simulink model "quad_control_elev8"  (Simulink 8.7)
settings: Solver=FixedStepAuto  StartTime=0.0  StopTime=20  FixedStep=0.01  RelTol=1e-3
InitFcn:
  | % --- Inner loop gains --------
  | Kp_pitch = 2.5;Ki_pitch = 0.005;Kd_pitch = 0.5;
  | 
  | Kp_roll = 2.5;Ki_roll = 0.005;Kd_roll = 0.5;
  | 
  | Kp_yaw = 10;Ki_yaw = 0.003;Kd_yaw = 2;
  | % --------------------------
  | 
  | % --- Outer loop gains --------
  | %P_X = 3.25; I_X = 0.45; D_X = 2;
  | %P_Y = 2.75; I_Y = 0.35; D_Y = 4.75;
  | %P_Z = 6; I_Z = 0.1; D_Z = 2;
  | 
  | %versoes 2
  | %P_X = 5;I_X = 0.1;D_X = 2.4;
  | %P_Y = 5;I_Y = 0.1;D_Y = 2.8;;
  | %P_Z = 32I_Z = 0.5;D_Z = 5;
  | 
  | %versoes CARLA
  | P_X = 9.44;I_X = 0.23;D_X = 2.36;
  | P_Y = 9.33;I_Y = 0.18;D_Y = 1.54;
  | P_Z = 28.09;I_Z = 5.65;D_Z = 16.16;
  | 
  | % --------------------------
  | 
  | % --- Saturation limits --------
  | attit_upper_limit = 10;
  | attit_lower_limit = -10;
  | 
  | pos_upper_limit = 1;
  | pos_lower_limit = -1;
  | 
  | mvel_upper_limit = 30;
  | mvel_lower_limit = 5;
  | % --------------------------
  | 
  | %gera o valor do angulo
  | %aleatoreamente para o treinamendo
  | %de posicao
  | rand_ang = pi + (-pi-pi).*rand(1,1);
  | rand_altur = 1 + (3-1).*rand(1,1);
  | 
  | global clientID;
  | clientID=-1;
undefined symbols (not defined in the file or in its folder): Angular, Linear, sigbuilder_block
libraries: simulink_extras x4, dspsigops x4, robotlib x3, aerolibtransform2 x1
settings Model: Creator=kleber  LastModifiedBy=kleber
settings DataIOCC: LimitDataPoints=off
settings DebuggingCC: UnderspecifiedInitializationDetection=Simplified  MergeDetectMultiDrivingBlocksExec=error  SolverPrmCheckMsg=warning
settings ConfigComp: CovSFcnEnable=off

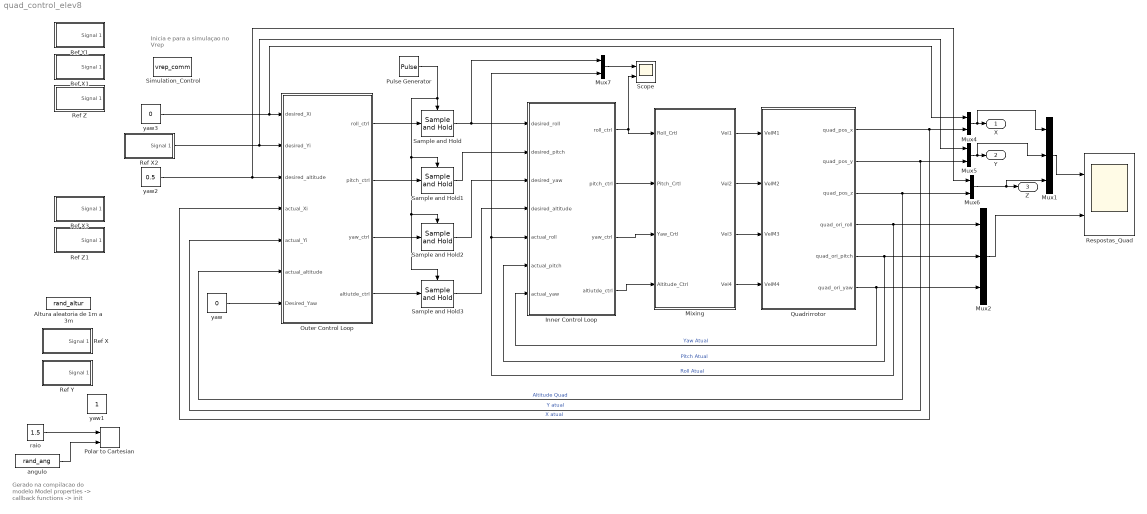
== system quad_control_elev8 ==
  note: Gerado na compilacao do modelo
      | Model properties -> callback functions
      | -> init
  note: Inicia e para a simulaçao no Vrep
  Altura aleatoria de 1m a 3m : Constant  Value=rand_altur
  Inner Control Loop : Subsystem
  Mixing : Subsystem
  Mux1 : Mux  Inputs=3
  Mux2 : Mux  Inputs=3
  Mux{4..7} (4 alike) : Mux  Inputs=2
  Outer Control Loop : Subsystem
  Polar to Cartesian : simulink_extras/Transformations/Polar to Cartesian
  Pulse Generator : DiscretePulseGenerator  PulseType=Time based  Period=0.1  PulseWidth=10
  Quadrirrotor : Subsystem
  Ref X : Subsystem  Tag=STV Subsys  LoadFcn=sigbuilder_block('load');  StartFcn=sigbuilder_block('start');  StopFcn=sigbuilder_block('stop');  ClipboardFcn=sigbuilder_block('clipboard');  mask(Sigbuilder block){}
      mask help: Sigbuilder GUI
      mask init:
      | if ~strcmp(get_param(bdroot(gcbh),'SimulationStatus'),'stopped') tuvar = sigbuilder_block('maskInit'); end
      settings: CopyFcn=sigbuilder_block('copy');  DeleteFcn=sigbuilder_block('delete');  ModelCloseFcn=sigbuilder_block('modelClose');  PreSaveFcn=sigbuilder_block('preSave');  PauseFcn=sigbuilder_block('pause')  ContinueFcn=sigbuilder_block('continue')  NameChangeFcn=sigbuilder_block('namechange');  OpenFcn=sigbuilder_block('open',[203.25 96 550.5 399.75 ]);  CloseFcn=sigbuilder_block('close');
      mask Display: plot(0,0,100,100,[10,10,40,40,10],[80,20,20,80,80],[40,10],[50,50], [40,27,10],[65,72,56],[40,25,25,10],[28,28,43,43]);
  Ref X1 : Subsystem  Tag=STV Subsys  LoadFcn=sigbuilder_block('load');  StartFcn=sigbuilder_block('start');  StopFcn=sigbuilder_block('stop');  ClipboardFcn=sigbuilder_block('clipboard');  mask(Sigbuilder block){}
      mask help: Sigbuilder GUI
      mask init:
      | if ~strcmp(get_param(bdroot(gcbh),'SimulationStatus'),'stopped') tuvar = sigbuilder_block('maskInit'); end
      settings: CopyFcn=sigbuilder_block('copy');  DeleteFcn=sigbuilder_block('delete');  ModelCloseFcn=sigbuilder_block('modelClose');  PreSaveFcn=sigbuilder_block('preSave');  PauseFcn=sigbuilder_block('pause')  ContinueFcn=sigbuilder_block('continue')  NameChangeFcn=sigbuilder_block('namechange');  OpenFcn=sigbuilder_block('open',[506.25 54.75 518.25 224.25 ]);  CloseFcn=sigbuilder_block('close');
      mask Display: plot(0,0,100,100,[10,10,40,40,10],[80,20,20,80,80],[40,10],[50,50], [40,27,10],[65,72,56],[40,25,25,10],[28,28,43,43]);
  Ref X2 : Subsystem  Tag=STV Subsys  LoadFcn=sigbuilder_block('load');  StartFcn=sigbuilder_block('start');  StopFcn=sigbuilder_block('stop');  ClipboardFcn=sigbuilder_block('clipboard');  mask(Sigbuilder block){}
      mask help: Sigbuilder GUI
      mask init:
      | if ~strcmp(get_param(bdroot(gcbh),'SimulationStatus'),'stopped') tuvar = sigbuilder_block('maskInit'); end
      settings: CopyFcn=sigbuilder_block('copy');  DeleteFcn=sigbuilder_block('delete');  ModelCloseFcn=sigbuilder_block('modelClose');  PreSaveFcn=sigbuilder_block('preSave');  PauseFcn=sigbuilder_block('pause')  ContinueFcn=sigbuilder_block('continue')  NameChangeFcn=sigbuilder_block('namechange');  OpenFcn=sigbuilder_block('open',[39.75 0 984.75 428.25 ]);  CloseFcn=sigbuilder_block('close');
      mask Display: plot(0,0,100,100,[10,10,40,40,10],[80,20,20,80,80],[40,10],[50,50], [40,27,10],[65,72,56],[40,25,25,10],[28,28,43,43]);
  Ref X3 : Subsystem  Tag=STV Subsys  LoadFcn=sigbuilder_block('load');  StartFcn=sigbuilder_block('start');  StopFcn=sigbuilder_block('stop');  ClipboardFcn=sigbuilder_block('clipboard');  mask(Sigbuilder block){}
      mask help: Sigbuilder GUI
      mask init:
      | if ~strcmp(get_param(bdroot(gcbh),'SimulationStatus'),'stopped') tuvar = sigbuilder_block('maskInit'); end
      settings: CopyFcn=sigbuilder_block('copy');  DeleteFcn=sigbuilder_block('delete');  ModelCloseFcn=sigbuilder_block('modelClose');  PreSaveFcn=sigbuilder_block('preSave');  PauseFcn=sigbuilder_block('pause')  ContinueFcn=sigbuilder_block('continue')  NameChangeFcn=sigbuilder_block('namechange');  OpenFcn=sigbuilder_block('open',[39.75 -17.25 984.75 495.75 ]);  CloseFcn=sigbuilder_block('close');
      mask Display: plot(0,0,100,100,[10,10,40,40,10],[80,20,20,80,80],[40,10],[50,50], [40,27,10],[65,72,56],[40,25,25,10],[28,28,43,43]);
  Ref Y : Subsystem  Tag=STV Subsys  LoadFcn=sigbuilder_block('load');  StartFcn=sigbuilder_block('start');  StopFcn=sigbuilder_block('stop');  ClipboardFcn=sigbuilder_block('clipboard');  mask(Sigbuilder block){}
      mask help: Sigbuilder GUI
      mask init:
      | if ~strcmp(get_param(bdroot(gcbh),'SimulationStatus'),'stopped') tuvar = sigbuilder_block('maskInit'); end
      settings: CopyFcn=sigbuilder_block('copy');  DeleteFcn=sigbuilder_block('delete');  ModelCloseFcn=sigbuilder_block('modelClose');  PreSaveFcn=sigbuilder_block('preSave');  PauseFcn=sigbuilder_block('pause')  ContinueFcn=sigbuilder_block('continue')  NameChangeFcn=sigbuilder_block('namechange');  OpenFcn=sigbuilder_block('open',[276 138 550.5 399.75 ]);  CloseFcn=sigbuilder_block('close');
      mask Display: plot(0,0,100,100,[10,10,40,40,10],[80,20,20,80,80],[40,10],[50,50], [40,27,10],[65,72,56],[40,25,25,10],[28,28,43,43]);
  Ref Y1 : Subsystem  Tag=STV Subsys  LoadFcn=sigbuilder_block('load');  StartFcn=sigbuilder_block('start');  StopFcn=sigbuilder_block('stop');  ClipboardFcn=sigbuilder_block('clipboard');  mask(Sigbuilder block){}
      mask help: Sigbuilder GUI
      mask init:
      | if ~strcmp(get_param(bdroot(gcbh),'SimulationStatus'),'stopped') tuvar = sigbuilder_block('maskInit'); end
      settings: CopyFcn=sigbuilder_block('copy');  DeleteFcn=sigbuilder_block('delete');  ModelCloseFcn=sigbuilder_block('modelClose');  PreSaveFcn=sigbuilder_block('preSave');  PauseFcn=sigbuilder_block('pause')  ContinueFcn=sigbuilder_block('continue')  NameChangeFcn=sigbuilder_block('namechange');  OpenFcn=sigbuilder_block('open',[270.75 145.5 510.75 222 ]);  CloseFcn=sigbuilder_block('close');
      mask Display: plot(0,0,100,100,[10,10,40,40,10],[80,20,20,80,80],[40,10],[50,50], [40,27,10],[65,72,56],[40,25,25,10],[28,28,43,43]);
  Ref Z : Subsystem  Tag=STV Subsys  LoadFcn=sigbuilder_block('load');  StartFcn=sigbuilder_block('start');  StopFcn=sigbuilder_block('stop');  ClipboardFcn=sigbuilder_block('clipboard');  mask(Sigbuilder block){}
      mask help: Sigbuilder GUI
      mask init:
      | if ~strcmp(get_param(bdroot(gcbh),'SimulationStatus'),'stopped') tuvar = sigbuilder_block('maskInit'); end
      settings: CopyFcn=sigbuilder_block('copy');  DeleteFcn=sigbuilder_block('delete');  ModelCloseFcn=sigbuilder_block('modelClose');  PreSaveFcn=sigbuilder_block('preSave');  PauseFcn=sigbuilder_block('pause')  ContinueFcn=sigbuilder_block('continue')  NameChangeFcn=sigbuilder_block('namechange');  OpenFcn=sigbuilder_block('open',[265.5 1.5 525.75 179.25 ]);  CloseFcn=sigbuilder_block('close');
      mask Display: plot(0,0,100,100,[10,10,40,40,10],[80,20,20,80,80],[40,10],[50,50], [40,27,10],[65,72,56],[40,25,25,10],[28,28,43,43]);
  Ref Z1 : Subsystem  Tag=STV Subsys  LoadFcn=sigbuilder_block('load');  StartFcn=sigbuilder_block('start');  StopFcn=sigbuilder_block('stop');  ClipboardFcn=sigbuilder_block('clipboard');  mask(Sigbuilder block){}
      mask help: Sigbuilder GUI
      mask init:
      | if ~strcmp(get_param(bdroot(gcbh),'SimulationStatus'),'stopped') tuvar = sigbuilder_block('maskInit'); end
      settings: CopyFcn=sigbuilder_block('copy');  DeleteFcn=sigbuilder_block('delete');  ModelCloseFcn=sigbuilder_block('modelClose');  PreSaveFcn=sigbuilder_block('preSave');  PauseFcn=sigbuilder_block('pause')  ContinueFcn=sigbuilder_block('continue')  NameChangeFcn=sigbuilder_block('namechange');  OpenFcn=sigbuilder_block('open',[58.5 0 966 213.75 ]);  CloseFcn=sigbuilder_block('close');
      mask Display: plot(0,0,100,100,[10,10,40,40,10],[80,20,20,80,80],[40,10],[50,50], [40,27,10],[65,72,56],[40,25,25,10],[28,28,43,43]);
  Respostas_Quad : Scope  NumInputPorts=2
  Sample and Hold{,1..3} (4 alike) : dspsigops/Sample and Hold  trig=Rising edge  initCond=0  latchinput=off
  Scope : Scope  NumInputPorts=2
  Simulation_Control : S-Function  FunctionName=vrep_comm  SFunctionDeploymentMode=off  EnableBusSupport=off
  angulo : Constant  Value=rand_ang
  raio : Constant  Value=1.5
  yaw : Constant  Value=0
  yaw1 : Constant
  yaw2 : Constant  Value=0.5
  yaw3 : Constant  Value=0
  X : Outport
  Y : Outport  Port=2
  Z : Outport  Port=3
  wires:
  Mux1/1 -> Respostas_Quad/1
  Mux2/1 -> Respostas_Quad/2
  Quadrirrotor/5(quad_ori_pitch) -> Inner Control Loop/6(actual_pitch), Mux2/2  "Pitch Atual"
  Quadrirrotor/4(quad_ori_roll) -> Mux7/2, Inner Control Loop/5(actual_roll), Mux2/1  "Roll Atual"
  Quadrirrotor/1(quad_pos_x) -> Outer Control Loop/4(actual_Xi), Mux4/2  "X atual"
  Quadrirrotor/3(quad_pos_z) -> Mux6/2, Outer Control Loop/6(actual_altitude)  "Altitude Quad"
  Quadrirrotor/6(quad_ori_yaw) -> Inner Control Loop/7(actual_yaw), Mux2/3  "Yaw Atual"
  Inner Control Loop/4(altiutde_ctrl) -> Mixing/4(Altitude_Ctrl)
  Sample and Hold3/1 -> Inner Control Loop/4(desired_altitude)
  Sample and Hold2/1 -> Inner Control Loop/3(desired_yaw)
  angulo/1 -> Polar to Cartesian/2
  raio/1 -> Polar to Cartesian/1
  yaw/1 -> Outer Control Loop/7(Desired_Yaw)
  Mux7/1 -> Scope/1
  Pulse Generator/1 -> Sample and Hold2/Trigger, Sample and Hold3/Trigger, Sample and Hold1/Trigger, Sample and Hold/Trigger
  Sample and Hold/1 -> Mux7/1, Inner Control Loop/1(desired_roll)
  Sample and Hold1/1 -> Inner Control Loop/2(desired_pitch)
  Outer Control Loop/4(altiutde_ctrl) -> Sample and Hold3/1
  Mux4/1 -> Mux1/1, X/1
  Mux5/1 -> Mux1/2, Y/1
  Mux6/1 -> Mux1/3, Z/1
  Ref X2/1(Signal 1) -> Mux5/1, Outer Control Loop/2(desired_Yi)
  yaw3/1 -> Mux4/1, Outer Control Loop/1(desired_Xi)
  yaw2/1 -> Mux6/1, Outer Control Loop/3(desired_altitude)
  Quadrirrotor/2(quad_pos_y) -> Outer Control Loop/5(actual_Yi), Mux5/2  "Y atual"
  Inner Control Loop/1(roll_ctrl) -> Mixing/1(Roll_Crtl), Scope/2
  Inner Control Loop/2(pitch_ctrl) -> Mixing/2(Pitch_Crtl)
  Inner Control Loop/3(yaw_ctrl) -> Mixing/3(Yaw_Crtl)
  Mixing/3(Vel3) -> Quadrirrotor/3(VelM3)
  Mixing/2(Vel2) -> Quadrirrotor/2(VelM2)
  Mixing/1(Vel1) -> Quadrirrotor/1(VelM1)
  Mixing/4(Vel4) -> Quadrirrotor/4(VelM4)
  Outer Control Loop/1(roll_ctrl) -> Sample and Hold/1
  Outer Control Loop/2(pitch_ctrl) -> Sample and Hold1/1
  Outer Control Loop/3(yaw_ctrl) -> Sample and Hold2/1

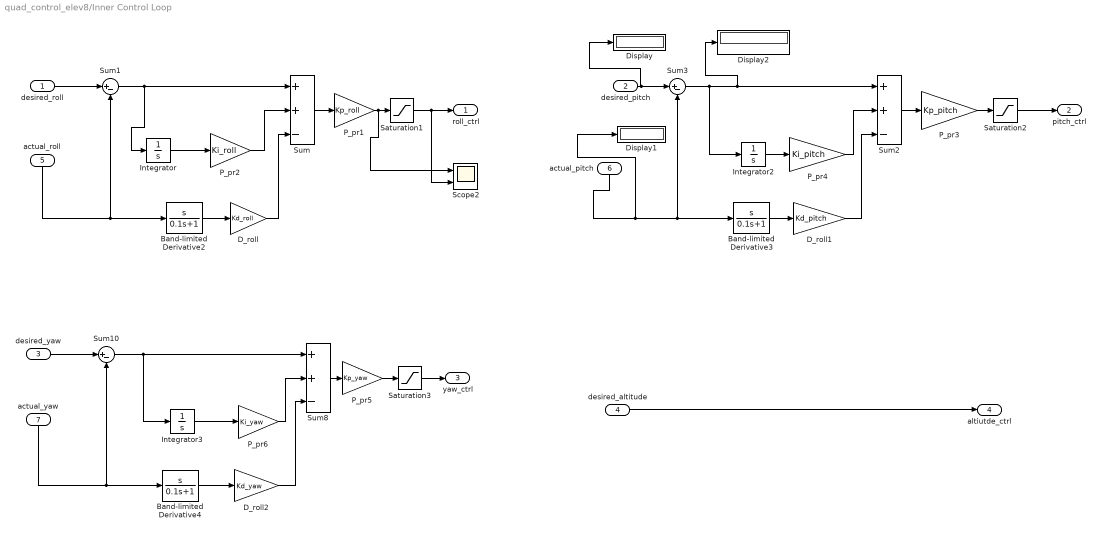
== system quad_control_elev8/Inner Control Loop ==
  desired_roll : Inport
  desired_pitch : Inport  Port=2
  desired_yaw : Inport  Port=3
  desired_altitude : Inport  Port=4
  actual_roll : Inport  Port=5
  actual_pitch : Inport  Port=6
  actual_yaw : Inport  Port=7
  Band-limited Derivative2 : TransferFcn  Numerator=[1 0]  Denominator=[0.1 1]
  Band-limited Derivative3 : TransferFcn  Numerator=[1 0]  Denominator=[0.1 1]
  Band-limited Derivative4 : TransferFcn  Numerator=[1 0]  Denominator=[0.1 1]
  D_roll : Gain  Gain=Kd_roll
  D_roll1 : Gain  Gain=Kd_pitch
  D_roll2 : Gain  Gain=Kd_yaw
  Display : Display
      settings: Decimation=3
  Display1 : Display
      settings: Decimation=3
  Display2 : Display
      settings: Decimation=3
  Integrator : Integrator
  Integrator2 : Integrator
  Integrator3 : Integrator
  P_pr1 : Gain  Gain=Kp_roll
  P_pr2 : Gain  Gain=Ki_roll
  P_pr3 : Gain  Gain=Kp_pitch
  P_pr4 : Gain  Gain=Ki_pitch
  P_pr5 : Gain  Gain=Kp_yaw
  P_pr6 : Gain  Gain=Ki_yaw
  Saturation1 : Saturate  UpperLimit=attit_upper_limit  LowerLimit=attit_lower_limit
  Saturation2 : Saturate  UpperLimit=attit_upper_limit  LowerLimit=attit_lower_limit
  Saturation3 : Saturate  UpperLimit=attit_upper_limit  LowerLimit=attit_lower_limit
  Scope2 : Scope  NumInputPorts=2
  Sum : Sum  Inputs=++-
  Sum1 : Sum  Inputs=|+-
  Sum10 : Sum  Inputs=|+-
  Sum2 : Sum  Inputs=++-
  Sum3 : Sum  Inputs=|+-
  Sum8 : Sum  Inputs=++-
  roll_ctrl : Outport
  pitch_ctrl : Outport  Port=2
  yaw_ctrl : Outport  Port=3
  altiutde_ctrl : Outport  Port=4
  wires:
  desired_altitude/1 -> altiutde_ctrl/1
  desired_roll/1 -> Sum1/1
  Sum1/1 -> Integrator/1, Sum/1
  Integrator/1 -> P_pr2/1
  actual_roll/1 -> Sum1/2, Band-limited Derivative2/1
  Band-limited Derivative2/1 -> D_roll/1
  desired_pitch/1 -> Display/1, Sum3/1
  Sum3/1 -> Sum2/1, Display2/1, Integrator2/1
  Integrator2/1 -> P_pr4/1
  actual_pitch/1 -> Sum3/2, Band-limited Derivative3/1, Display1/1
  Band-limited Derivative3/1 -> D_roll1/1
  desired_yaw/1 -> Sum10/1
  Sum10/1 -> Sum8/1, Integrator3/1
  Integrator3/1 -> P_pr6/1
  actual_yaw/1 -> Sum10/2, Band-limited Derivative4/1
  Band-limited Derivative4/1 -> D_roll2/1
  Saturation1/1 -> roll_ctrl/1, Scope2/2
  Saturation3/1 -> yaw_ctrl/1
  Saturation2/1 -> pitch_ctrl/1
  Sum/1 -> P_pr1/1
  P_pr1/1 -> Scope2/1, Saturation1/1
  D_roll/1 -> Sum/3
  D_roll1/1 -> Sum2/3
  Sum2/1 -> P_pr3/1
  P_pr3/1 -> Saturation2/1
  Sum8/1 -> P_pr5/1
  P_pr5/1 -> Saturation3/1
  D_roll2/1 -> Sum8/3
  P_pr2/1 -> Sum/2
  P_pr4/1 -> Sum2/2
  P_pr6/1 -> Sum8/2

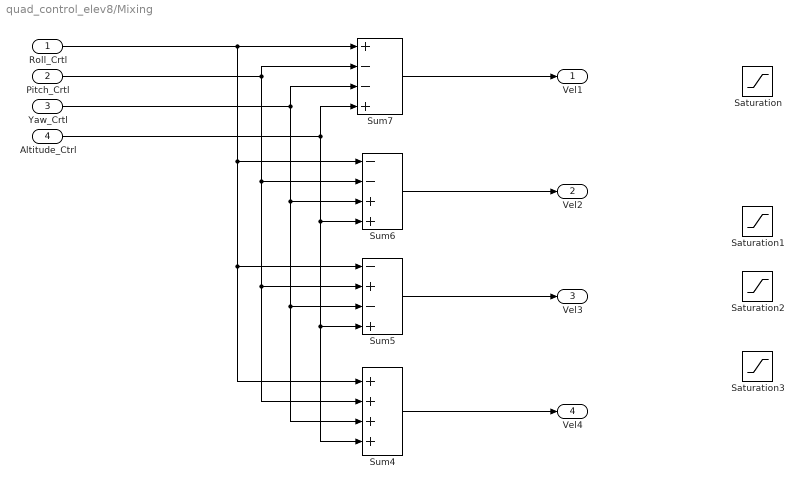
== system quad_control_elev8/Mixing ==
  Roll_Crtl : Inport
  Pitch_Crtl : Inport  Port=2
  Yaw_Crtl : Inport  Port=3
  Altitude_Ctrl : Inport  Port=4
  Saturation{,1..3} (4 alike) : Saturate  UpperLimit=mvel_upper_limit  LowerLimit=mvel_lower_limit
  Sum4 : Sum  Inputs=++++
  Sum5 : Sum  Inputs=-+-+
  Sum6 : Sum  Inputs=--++
  Sum7 : Sum  Inputs=+--+
  Vel1 : Outport
  Vel2 : Outport  Port=2
  Vel3 : Outport  Port=3
  Vel4 : Outport  Port=4
  wires:
  Yaw_Crtl/1 -> Sum4/3, Sum5/3, Sum6/3, Sum7/3
  Roll_Crtl/1 -> Sum4/1, Sum5/1, Sum6/1, Sum7/1
  Pitch_Crtl/1 -> Sum4/2, Sum5/2, Sum6/2, Sum7/2
  Altitude_Ctrl/1 -> Sum4/4, Sum5/4, Sum6/4, Sum7/4
  Sum7/1 -> Vel1/1
  Sum6/1 -> Vel2/1
  Sum5/1 -> Vel3/1
  Sum4/1 -> Vel4/1

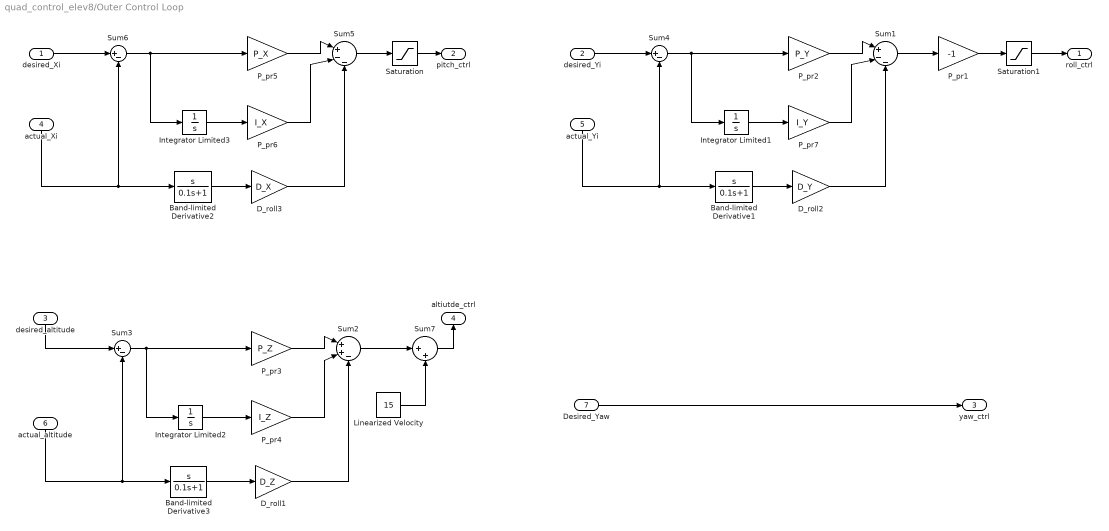
== system quad_control_elev8/Outer Control Loop ==
  desired_Xi : Inport
  desired_Yi : Inport  Port=2
  desired_altitude : Inport  Port=3
  actual_Xi : Inport  Port=4
  actual_Yi : Inport  Port=5
  actual_altitude : Inport  Port=6
  Desired_Yaw : Inport  Port=7
  Band-limited Derivative1 : TransferFcn  Numerator=[1 0]  Denominator=[0.1 1]
  Band-limited Derivative2 : TransferFcn  Numerator=[1 0]  Denominator=[0.1 1]
  Band-limited Derivative3 : TransferFcn  Numerator=[1 0]  Denominator=[0.1 1]
  D_roll1 : Gain  Gain=D_Z
  D_roll2 : Gain  Gain=D_Y
  D_roll3 : Gain  Gain=D_X
  Integrator Limited1 : Integrator  LimitOutput=on  UpperSaturationLimit=0.5  LowerSaturationLimit=-0.5
  Integrator Limited2 : Integrator  LimitOutput=on  UpperSaturationLimit=1  LowerSaturationLimit=0
  Integrator Limited3 : Integrator  LimitOutput=on  UpperSaturationLimit=0.5  LowerSaturationLimit=-0.5
  Linearized Velocity : Constant  Value=15
  P_pr1 : Gain  Gain=-1
  P_pr2 : Gain  Gain=P_Y
  P_pr3 : Gain  Gain=P_Z
  P_pr4 : Gain  Gain=I_Z
  P_pr5 : Gain  Gain=P_X
  P_pr6 : Gain  Gain=I_X
  P_pr7 : Gain  Gain=I_Y
  Saturation : Saturate  UpperLimit=2  LowerLimit=-2
  Saturation1 : Saturate  UpperLimit=2  LowerLimit=-2
  Sum1 : Sum  Inputs=|+--
  Sum2 : Sum  Inputs=|++-
  Sum3 : Sum  Inputs=|+-
  Sum4 : Sum  Inputs=|+-
  Sum5 : Sum  Inputs=|+--
  Sum6 : Sum  Inputs=|+-
  Sum7 : Sum  Inputs=|++
  roll_ctrl : Outport
  pitch_ctrl : Outport  Port=2
  yaw_ctrl : Outport  Port=3
  altiutde_ctrl : Outport  Port=4
  wires:
  Sum3/1 -> Integrator Limited2/1, P_pr3/1
  Integrator Limited2/1 -> P_pr4/1
  P_pr3/1 -> Sum2/1
  P_pr4/1 -> Sum2/2
  D_roll1/1 -> Sum2/3
  actual_altitude/1 -> Sum3/2, Band-limited Derivative3/1
  Band-limited Derivative3/1 -> D_roll1/1
  desired_altitude/1 -> Sum3/1
  Sum7/1 -> altiutde_ctrl/1
  Desired_Yaw/1 -> yaw_ctrl/1
  Sum6/1 -> Integrator Limited3/1, P_pr5/1
  Integrator Limited3/1 -> P_pr6/1
  P_pr5/1 -> Sum5/1
  D_roll3/1 -> Sum5/3
  actual_Xi/1 -> Band-limited Derivative2/1, Sum6/2
  Band-limited Derivative2/1 -> D_roll3/1
  desired_Xi/1 -> Sum6/1
  P_pr6/1 -> Sum5/2
  Sum4/1 -> Integrator Limited1/1, P_pr2/1
  Integrator Limited1/1 -> P_pr7/1
  P_pr2/1 -> Sum1/1
  D_roll2/1 -> Sum1/3
  actual_Yi/1 -> Band-limited Derivative1/1, Sum4/2
  Band-limited Derivative1/1 -> D_roll2/1
  desired_Yi/1 -> Sum4/1
  P_pr7/1 -> Sum1/2
  Sum1/1 -> P_pr1/1
  Sum2/1 -> Sum7/1
  Linearized Velocity/1 -> Sum7/2
  Sum5/1 -> Saturation/1
  Saturation/1 -> pitch_ctrl/1
  P_pr1/1 -> Saturation1/1
  Saturation1/1 -> roll_ctrl/1

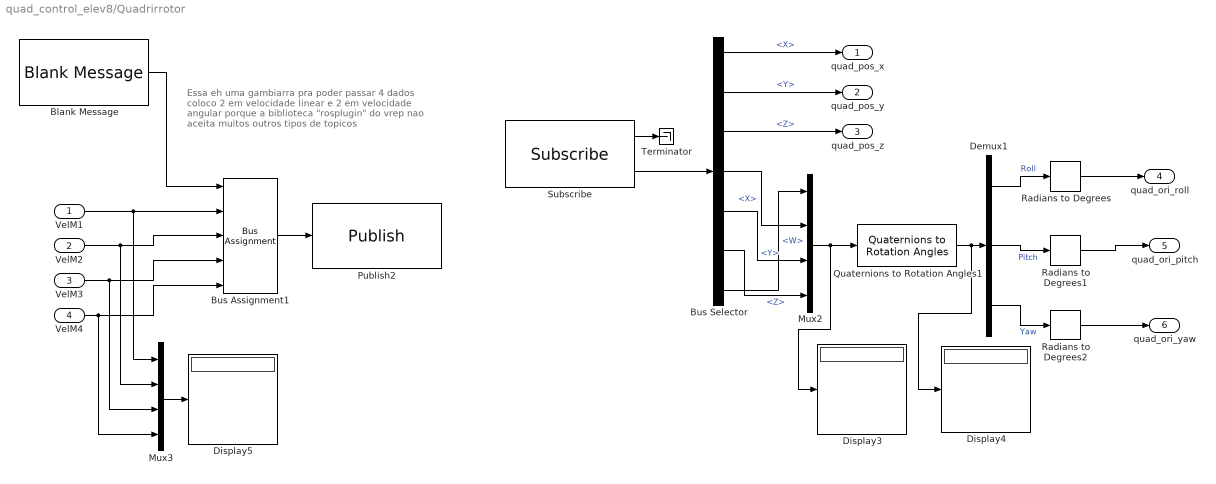
== system quad_control_elev8/Quadrirrotor ==
  note: Essa eh uma gambiarra pra poder passar 4 dados coloco 2 em velocidade linear e 2 em velocidade angular porque a biblioteca "rosplugin" do vrep nao aceita muitos outros tipos de topicos
  VelM1 : Inport
  VelM2 : Inport  Port=2
  VelM3 : Inport  Port=3
  VelM4 : Inport  Port=4
  Blank Message : robotlib/Blank Message  SourceLibraryInfo=This block requires Robotics System Toolbox  messageType=geometry_msgs/Twist  SampleTime=inf
  Bus Assignment1 : BusAssignment  DialogController=Simulink.DDGSource_BusAssignment  AssignedSignals=Linear.X,Linear.Y,Angular.X,Angular.Y
  Bus Selector : BusSelector  OutputSignals=Pose.Position.X,Pose.Position.Y,Pose.Position.Z,Pose.Orientation.X,Pose.Orientation.Y,Pose.Orientation.Z,Pose.Orientation.W
  Demux1 : Demux  Outputs=3
  Display3 : Display
  Display4 : Display
  Display5 : Display
  Mux2 : Mux
  Mux3 : Mux
  Publish2 : robotlib/Publish  SourceLibraryInfo=This block requires Robotics System Toolbox  topicSource=Select from ROS network  topic=/control_signals  messageType=geometry_msgs/Twist  messageQueueLength=105
  Quaternions to Rotation Angles1 : aerolibtransform2/Quaternions to Rotation Angles  rotationOrder=XYZ
  Radians to Degrees : simulink_extras/Transformations/Radians to Degrees
  Radians to Degrees1 : simulink_extras/Transformations/Radians to Degrees
  Radians to Degrees2 : simulink_extras/Transformations/Radians to Degrees
  Subscribe : robotlib/Subscribe  SourceLibraryInfo=This block requires Robotics System Toolbox  topicSource=Select from ROS network  topic=/quad_pos_ang  messageType=geometry_msgs/PoseStamped  sampleTime=-1  messageQueueLength=51
  Terminator : Terminator
  quad_pos_x : Outport
  quad_pos_y : Outport  Port=2
  quad_pos_z : Outport  Port=3
  quad_ori_roll : Outport  Port=4
  quad_ori_pitch : Outport  Port=5
  quad_ori_yaw : Outport  Port=6
  wires:
  VelM1/1 -> Mux3/1, Bus Assignment1/2
  Bus Selector/1 -> quad_pos_x/1  "<X>"
  Bus Selector/2 -> quad_pos_y/1  "<Y>"
  Bus Selector/3 -> quad_pos_z/1  "<Z>"
  Bus Assignment1/1 -> Publish2/1
  Blank Message/1 -> Bus Assignment1/1
  Subscribe/2 -> Bus Selector/1
  Subscribe/1 -> Terminator/1
  Bus Selector/5 -> Mux2/3  "<Y>"
  Bus Selector/6 -> Mux2/4  "<Z>"
  Bus Selector/7 -> Mux2/1  "<W>"
  Mux2/1 -> Quaternions to Rotation Angles1/1, Display3/1
  Bus Selector/4 -> Mux2/2  "<X>"
  VelM3/1 -> Mux3/3, Bus Assignment1/4
  VelM4/1 -> Mux3/4, Bus Assignment1/5
  Quaternions to Rotation Angles1/1 -> Display4/1, Demux1/1
  Mux3/1 -> Display5/1
  VelM2/1 -> Mux3/2, Bus Assignment1/3
  Radians to Degrees2/1 -> quad_ori_yaw/1
  Radians to Degrees1/1 -> quad_ori_pitch/1
  Radians to Degrees/1 -> quad_ori_roll/1
  Demux1/1 -> Radians to Degrees/1  "Roll"
  Demux1/2 -> Radians to Degrees1/1  "Pitch"
  Demux1/3 -> Radians to Degrees2/1  "Yaw"

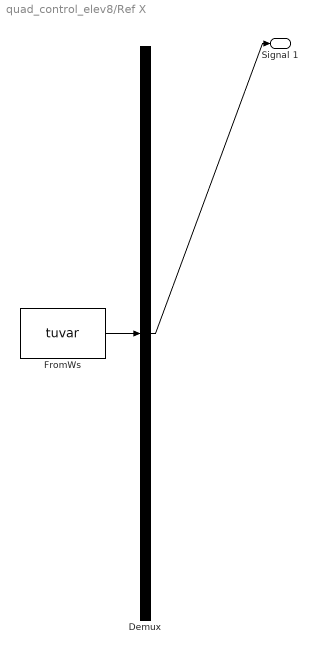
== system quad_control_elev8/Ref X ==
  Demux : Demux  Tag=STV Demux  Outputs=1
  FromWs : FromWorkspace  Tag=STV FromWs  VariableName=tuvar  SampleTime=0  SigBuilderData=DataTag0  VnvData=DataTag1
      SigBuilderData=|
      | common.afterFinalStr = 'Extrapolate'
      | common.sampleTime = 0
      | dataSet.timeRange = [0 50]
      | dataSet.name = 'Group 1'
      | sbobj.Name = 'Signal Builder'
      | sbobj.Groups.Name = 'Group 1'
      | sbobj.Groups.Signals.Name = 'Signal 1'
      | sbobj.Groups.Signals.XData = [0 5 25 30 50]
      | sbobj.Groups.Signals.YData = [0 1 1 0 0]
      | sbobj.Groups.TimeRange = [0 50]
  Signal 1 : Outport  Tag=STV Outport
  wires:
  FromWs/1 -> Demux/1
  Demux/1 -> Signal 1/1

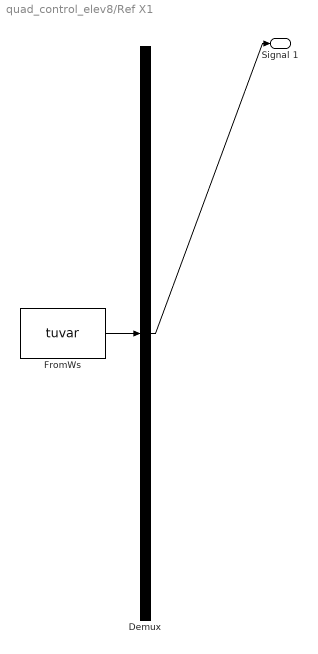
== system quad_control_elev8/Ref X1 ==
  Demux : Demux  Tag=STV Demux  Outputs=1
  FromWs : FromWorkspace  Tag=STV FromWs  VariableName=tuvar  SampleTime=0  SigBuilderData=DataTag2  VnvData=DataTag3
      SigBuilderData=|
      | common.afterFinalStr = 'Extrapolate'
      | common.sampleTime = 0
      | dataSet.timeRange = [0 200]
      | dataSet.name = 'Group 1'
      | sbobj.Name = 'Signal Builder'
      | sbobj.Groups.Name = 'Group 1'
      | sbobj.Groups.Signals.Name = 'Signal 1'
      | sbobj.Groups.Signals.XData = [0 10 100 110 200]
      | sbobj.Groups.Signals.YData = [0 1 1 1.5 1.5]
      | sbobj.Groups.TimeRange = [0 200]
  Signal 1 : Outport  Tag=STV Outport
  wires:
  FromWs/1 -> Demux/1
  Demux/1 -> Signal 1/1

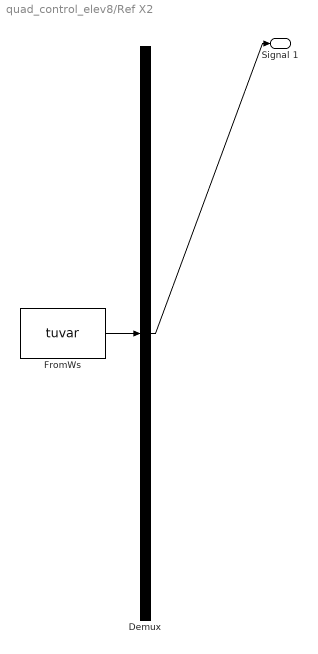
== system quad_control_elev8/Ref X2 ==
  Demux : Demux  Tag=STV Demux  Outputs=1
  FromWs : FromWorkspace  Tag=STV FromWs  VariableName=tuvar  SampleTime=0  SigBuilderData=DataTag4  VnvData=DataTag5
      SigBuilderData=|
      | common.afterFinalStr = 'Extrapolate'
      | common.sampleTime = 0
      | dataSet.timeRange = [0 250]
      | dataSet.name = 'Group 1'
      | sbobj.Name = 'Signal Builder'
      | sbobj.Groups.Name = 'Group 1'
      | sbobj.Groups.Signals.Name = 'Signal 1'
      | sbobj.Groups.Signals.XData = [0 50 100 250]
      | sbobj.Groups.Signals.YData = [0 0 2 2]
      | sbobj.Groups.TimeRange = [0 250]
  Signal 1 : Outport  Tag=STV Outport
  wires:
  Demux/1 -> Signal 1/1
  FromWs/1 -> Demux/1

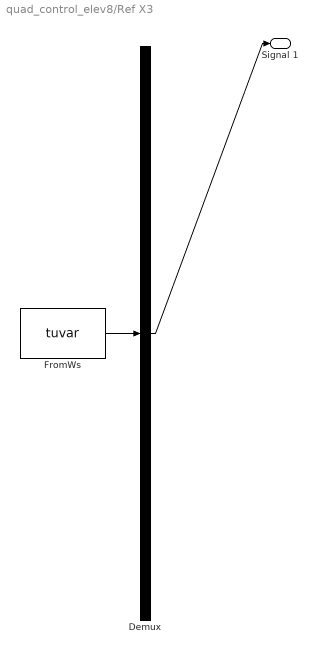
== system quad_control_elev8/Ref X3 ==
  Demux : Demux  Tag=STV Demux  Outputs=1
  FromWs : FromWorkspace  Tag=STV FromWs  VariableName=tuvar  SampleTime=0  SigBuilderData=DataTag6  VnvData=DataTag7
      SigBuilderData=|
      | common.afterFinalStr = 'Extrapolate'
      | common.sampleTime = 0
      | dataSet.timeRange = [0 250]
      | dataSet.name = 'Group 1'
      | sbobj.Name = 'Signal Builder'
      | sbobj.Groups.Name = 'Group 1'
      | sbobj.Groups.Signals.Name = 'Signal 1'
      | sbobj.Groups.Signals.XData = [0 50 70 250]
      | sbobj.Groups.Signals.YData = [0 0 2 2]
      | sbobj.Groups.TimeRange = [0 250]
  Signal 1 : Outport  Tag=STV Outport
  wires:
  FromWs/1 -> Demux/1
  Demux/1 -> Signal 1/1

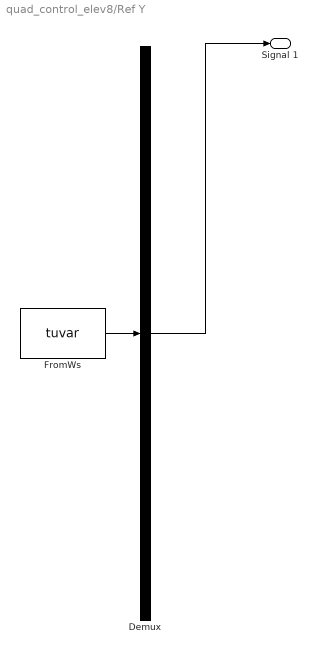
== system quad_control_elev8/Ref Y ==
  Demux : Demux  Tag=STV Demux  Outputs=1
  FromWs : FromWorkspace  Tag=STV FromWs  VariableName=tuvar  SampleTime=0  SigBuilderData=DataTag8  VnvData=DataTag9
      SigBuilderData=|
      | common.afterFinalStr = 'Extrapolate'
      | common.sampleTime = 0
      | dataSet.timeRange = [0 50]
      | dataSet.name = 'Group 1'
      | sbobj.Name = 'Signal Builder'
      | sbobj.Groups.Name = 'Group 1'
      | sbobj.Groups.Signals.Name = 'Signal 1'
      | sbobj.Groups.Signals.XData = [0 10 15 35 40 50]
      | sbobj.Groups.Signals.YData = [0 0 1 1 0 0]
      | sbobj.Groups.TimeRange = [0 50]
  Signal 1 : Outport  Tag=STV Outport
  wires:
  Demux/1 -> Signal 1/1
  FromWs/1 -> Demux/1

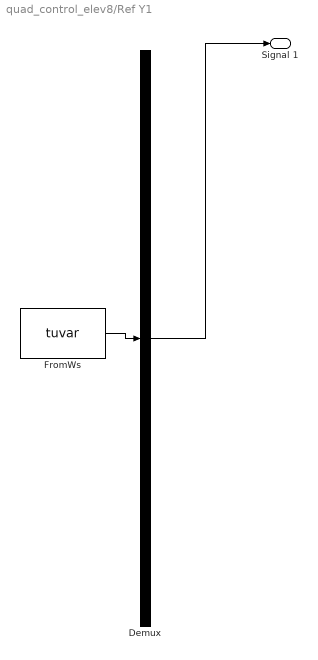
== system quad_control_elev8/Ref Y1 ==
  Demux : Demux  Tag=STV Demux  Outputs=1
  FromWs : FromWorkspace  Tag=STV FromWs  VariableName=tuvar  SampleTime=0  SigBuilderData=DataTag10  VnvData=DataTag11
      SigBuilderData=|
      | common.afterFinalStr = 'Extrapolate'
      | common.sampleTime = 0
      | dataSet.timeRange = [0 200]
      | dataSet.name = 'Group 1'
      | sbobj.Name = 'Signal Builder'
      | sbobj.Groups.Name = 'Group 1'
      | sbobj.Groups.Signals.Name = 'Signal 1'
      | sbobj.Groups.Signals.XData = [0 10 50 75 100 130 150 170 200]
      | sbobj.Groups.Signals.YData = [0 0.5 0.5 2.5 2.5 0.5 0.5 2.5 2.5]
      | sbobj.Groups.TimeRange = [0 200]
  Signal 1 : Outport  Tag=STV Outport
  wires:
  Demux/1 -> Signal 1/1
  FromWs/1 -> Demux/1

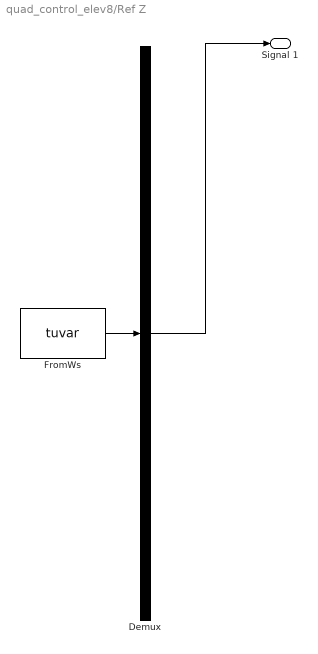
== system quad_control_elev8/Ref Z ==
  Demux : Demux  Tag=STV Demux  Outputs=1
  FromWs : FromWorkspace  Tag=STV FromWs  VariableName=tuvar  SampleTime=0  SigBuilderData=DataTag12  VnvData=DataTag13
      SigBuilderData=|
      | common.afterFinalStr = 'Extrapolate'
      | common.sampleTime = 0
      | dataSet.timeRange = [0 200]
      | dataSet.name = 'Group 1'
      | sbobj.Name = 'Signal Builder'
      | sbobj.Groups.Name = 'Group 1'
      | sbobj.Groups.Signals.Name = 'Signal 1'
      | sbobj.Groups.Signals.XData = [0 5 30 35 45 50 80 85 95 100 130 135 145 150 175 180 190 195 200]
      | sbobj.Groups.Signals.YData = [0 1 1 0.3 0.3 1 1 0.3 0.3 1 1 0.3 0.3 1 1 0.3 0.3 1 1]
      | sbobj.Groups.TimeRange = [0 200]
  Signal 1 : Outport  Tag=STV Outport
  wires:
  Demux/1 -> Signal 1/1
  FromWs/1 -> Demux/1

== system quad_control_elev8/Ref Z1 ==
  Demux : Demux  Tag=STV Demux  Outputs=1
  FromWs : FromWorkspace  Tag=STV FromWs  VariableName=tuvar  SampleTime=0  SigBuilderData=DataTag14  VnvData=DataTag15
      SigBuilderData=|
      | common.afterFinalStr = 'Extrapolate'
      | common.sampleTime = 0
      | dataSet.timeRange = [0 250]
      | dataSet.name = 'Group 1'
      | sbobj.Name = 'Signal Builder'
      | sbobj.Groups.Name = 'Group 1'
      | sbobj.Groups.Signals.Name = 'Signal 1'
      | sbobj.Groups.Signals.XData = [0 10 120 130 140 150 200 215 220 235 250]
      | sbobj.Groups.Signals.YData = [0.2 0.5 0.5 0.15 0.15 0.5 0.5 0.15 0.15 0.5 0.5]
      | sbobj.Groups.TimeRange = [0 250]
  Signal 1 : Outport  Tag=STV Outport
  wires:
  Demux/1 -> Signal 1/1
  FromWs/1 -> Demux/1
